simulink model "NoEngine"  (R2020a)
settings: configuration reference "Reference" (kept outside this file)
settings Model: DataDictionary=SystemDD_v4.sldd  Creator=koshiro
settings ConfigSetRef: SourceName=Reference

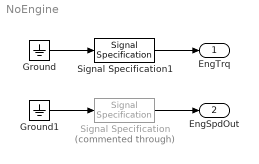
== system NoEngine ==
  Ground : Ground
  Ground1 : Ground
  Signal Specification : SignalSpecification  Commented=through  Unit=rev/min
  Signal Specification1 : SignalSpecification  Unit=N*m
  EngTrq : Outport
  EngSpdOut : Outport  Port=2
  wires:
  Ground/1 -> Signal Specification1/1
  Ground1/1 -> Signal Specification/1
  Signal Specification/1 -> EngSpdOut/1
  Signal Specification1/1 -> EngTrq/1
